simulink model "Aufg7_2"  (R2018a)
settings: Solver=VariableStepAuto  StartTime=0.0  StopTime=60  RelTol=1e-3
undefined symbols (not defined in the file or in its folder): des, gcbh
settings Model: Creator=Naveen  LastModifiedBy=Naveen
settings DataIOCC: ReturnWorkspaceOutputs=on
settings SFSimCC: SimUseLocalCustomCode=on
settings RTWCC: RTWUseLocalCustomCode=on

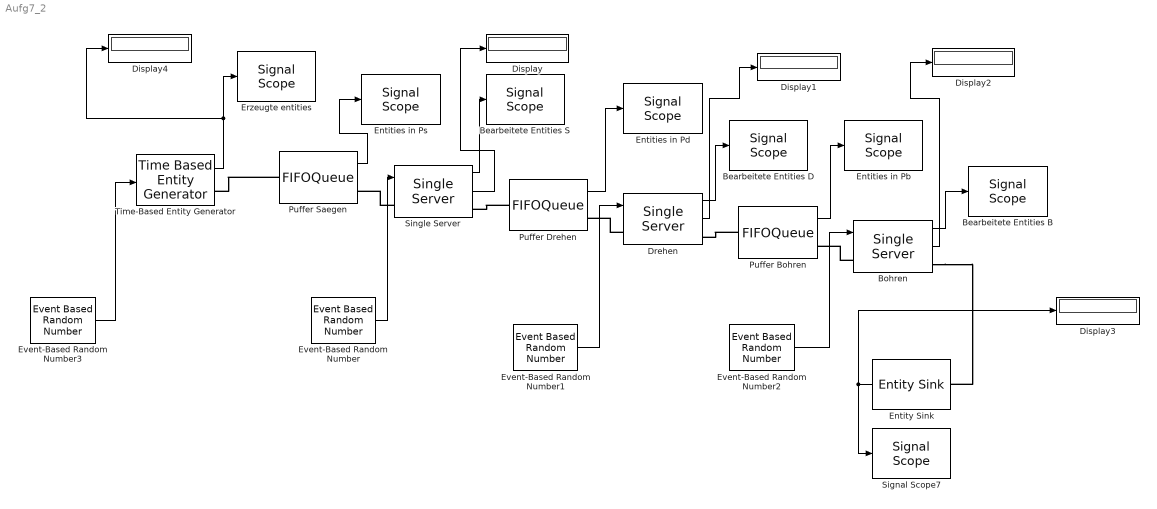
== system Aufg7_2 ==
  Bearbeitete Entities B : SignalScope  LoadFcn=des.scope.CallbackSupport('seLoadFcn',gcbh)  StartFcn=des.scope.CallbackSupport('seStartFcn',gcbh)  StopFcn=des.scope.CallbackSupport('seStopFcn',gcbh)
      settings: CopyFcn=des.scope.CallbackSupport('seCopyFcn',gcbh)  DeleteFcn=des.scope.CallbackSupport('seDeleteFcn',gcbh)  PreSaveFcn=des.scope.CallbackSupport('sePreSaveFcn',gcbh)  NameChangeFcn=des.scope.CallbackSupport('seNameChangeFcn',gcbh)  OpenFcn=des.scope.CallbackSupport('seOpenFcn',gcbh)
  Bearbeitete Entities D : SignalScope  LoadFcn=des.scope.CallbackSupport('seLoadFcn',gcbh)  StartFcn=des.scope.CallbackSupport('seStartFcn',gcbh)  StopFcn=des.scope.CallbackSupport('seStopFcn',gcbh)
      settings: CopyFcn=des.scope.CallbackSupport('seCopyFcn',gcbh)  DeleteFcn=des.scope.CallbackSupport('seDeleteFcn',gcbh)  PreSaveFcn=des.scope.CallbackSupport('sePreSaveFcn',gcbh)  NameChangeFcn=des.scope.CallbackSupport('seNameChangeFcn',gcbh)  OpenFcn=des.scope.CallbackSupport('seOpenFcn',gcbh)
  Bearbeitete Entities S : SignalScope  LoadFcn=des.scope.CallbackSupport('seLoadFcn',gcbh)  StartFcn=des.scope.CallbackSupport('seStartFcn',gcbh)  StopFcn=des.scope.CallbackSupport('seStopFcn',gcbh)
      settings: CopyFcn=des.scope.CallbackSupport('seCopyFcn',gcbh)  DeleteFcn=des.scope.CallbackSupport('seDeleteFcn',gcbh)  PreSaveFcn=des.scope.CallbackSupport('sePreSaveFcn',gcbh)  NameChangeFcn=des.scope.CallbackSupport('seNameChangeFcn',gcbh)  OpenFcn=des.scope.CallbackSupport('seOpenFcn',gcbh)
  Bohren : SingleServer  ServiceTimeFrom=Signal port t  ServiceTime=ts_bohr  StatNumberDeparted=on  StatUtilization=on
      settings: OutputPortMap=o0,o5
  Display{,1..4} (5 alike) : Display
  Drehen : SingleServer  ServiceTimeFrom=Signal port t  ServiceTime=ts_dreh  StatNumberDeparted=on  StatUtilization=on
      settings: OutputPortMap=o0,o5
  Entities in Pb : SignalScope  LoadFcn=des.scope.CallbackSupport('seLoadFcn',gcbh)  StartFcn=des.scope.CallbackSupport('seStartFcn',gcbh)  StopFcn=des.scope.CallbackSupport('seStopFcn',gcbh)
      settings: CopyFcn=des.scope.CallbackSupport('seCopyFcn',gcbh)  DeleteFcn=des.scope.CallbackSupport('seDeleteFcn',gcbh)  PreSaveFcn=des.scope.CallbackSupport('sePreSaveFcn',gcbh)  NameChangeFcn=des.scope.CallbackSupport('seNameChangeFcn',gcbh)  OpenFcn=des.scope.CallbackSupport('seOpenFcn',gcbh)
  Entities in Pd : SignalScope  LoadFcn=des.scope.CallbackSupport('seLoadFcn',gcbh)  StartFcn=des.scope.CallbackSupport('seStartFcn',gcbh)  StopFcn=des.scope.CallbackSupport('seStopFcn',gcbh)
      settings: CopyFcn=des.scope.CallbackSupport('seCopyFcn',gcbh)  DeleteFcn=des.scope.CallbackSupport('seDeleteFcn',gcbh)  PreSaveFcn=des.scope.CallbackSupport('sePreSaveFcn',gcbh)  NameChangeFcn=des.scope.CallbackSupport('seNameChangeFcn',gcbh)  OpenFcn=des.scope.CallbackSupport('seOpenFcn',gcbh)
  Entities in Ps : SignalScope  LoadFcn=des.scope.CallbackSupport('seLoadFcn',gcbh)  StartFcn=des.scope.CallbackSupport('seStartFcn',gcbh)  StopFcn=des.scope.CallbackSupport('seStopFcn',gcbh)
      settings: CopyFcn=des.scope.CallbackSupport('seCopyFcn',gcbh)  DeleteFcn=des.scope.CallbackSupport('seDeleteFcn',gcbh)  PreSaveFcn=des.scope.CallbackSupport('sePreSaveFcn',gcbh)  NameChangeFcn=des.scope.CallbackSupport('seNameChangeFcn',gcbh)  OpenFcn=des.scope.CallbackSupport('seOpenFcn',gcbh)
  Entity Sink : EntitySink  StatNumberArrived=on
  Erzeugte entities : SignalScope  LoadFcn=des.scope.CallbackSupport('seLoadFcn',gcbh)  StartFcn=des.scope.CallbackSupport('seStartFcn',gcbh)  StopFcn=des.scope.CallbackSupport('seStopFcn',gcbh)
      settings: CopyFcn=des.scope.CallbackSupport('seCopyFcn',gcbh)  DeleteFcn=des.scope.CallbackSupport('seDeleteFcn',gcbh)  PreSaveFcn=des.scope.CallbackSupport('sePreSaveFcn',gcbh)  NameChangeFcn=des.scope.CallbackSupport('seNameChangeFcn',gcbh)  OpenFcn=des.scope.CallbackSupport('seOpenFcn',gcbh)
  Event-Based Random Number : EventBasedRandomNumber  Distribution=Uniform  minUnif=0.3  maxUnif=1.7
  Event-Based Random Number1 : EventBasedRandomNumber  Distribution=Triangular  minTri=0.5
  Event-Based Random Number2 : EventBasedRandomNumber  Distribution=Uniform  minUnif=0.3  maxUnif=0.7
  Event-Based Random Number3 : EventBasedRandomNumber  minUnif=0.3  maxUnif=1.7
  Puffer Bohren : FIFOQueue  Capacity=inf  StatNumberInBlock=on
      settings: OutputPortMap=o1
  Puffer Drehen : FIFOQueue  Capacity=10  StatNumberInBlock=on
      settings: OutputPortMap=o1
  Puffer Saegen : FIFOQueue  Capacity=inf  StatNumberInBlock=on
      settings: OutputPortMap=o1
  Signal Scope7 : SignalScope  LoadFcn=des.scope.CallbackSupport('seLoadFcn',gcbh)  StartFcn=des.scope.CallbackSupport('seStartFcn',gcbh)  StopFcn=des.scope.CallbackSupport('seStopFcn',gcbh)
      settings: CopyFcn=des.scope.CallbackSupport('seCopyFcn',gcbh)  DeleteFcn=des.scope.CallbackSupport('seDeleteFcn',gcbh)  PreSaveFcn=des.scope.CallbackSupport('sePreSaveFcn',gcbh)  NameChangeFcn=des.scope.CallbackSupport('seNameChangeFcn',gcbh)  OpenFcn=des.scope.CallbackSupport('seOpenFcn',gcbh)
  Single Server : SingleServer  ServiceTimeFrom=Signal port t  ServiceTime=ts_sage  StatNumberDeparted=on  StatUtilization=on
      settings: OutputPortMap=o0,o5
  Time-Based Entity Generator : TimeBasedEntityGenerator  GenerateEntitiesUpon=Intergeneration time from port t  StatNumberDeparted=on
  wires:
  Drehen/2 -> Display1/1
  Bohren/2 -> Display2/1
  Single Server/2 -> Display/1
  Entity Sink/1 -> Signal Scope7/1, Display3/1
  Time-Based Entity Generator/1 -> Display4/1, Erzeugte entities/1
  Bohren/1 -> Bearbeitete Entities B/1
  Puffer Bohren/1 -> Entities in Pb/1
  Drehen/1 -> Bearbeitete Entities D/1
  Puffer Drehen/1 -> Entities in Pd/1
  Single Server/1 -> Bearbeitete Entities S/1
  Puffer Saegen/1 -> Entities in Ps/1
  Event-Based Random Number/1 -> Single Server/1
  Event-Based Random Number1/1 -> Drehen/1
  Event-Based Random Number2/1 -> Bohren/1
  Event-Based Random Number3/1 -> Time-Based Entity Generator/1
  connections:
  Puffer Drehen/LConn1 -- Single Server/RConn1
  Drehen/LConn1 -- Puffer Drehen/RConn1
  Single Server/LConn1 -- Puffer Saegen/RConn1
  Puffer Saegen/LConn1 -- Time-Based Entity Generator/RConn1
  Puffer Bohren/LConn1 -- Drehen/RConn1
  Bohren/LConn1 -- Puffer Bohren/RConn1
  Bohren/RConn1 -- Entity Sink/LConn1
